simulink model "sedemo_mm1"  (Simulink 7.5)
settings: Solver=ode45  StartTime=0.0  StopTime=10000  RelTol=1e-3
PostLoadFcn:
  | open_system([gcs '/Arrival Rate Gain']);
undefined symbols (not defined in the file or in its folder): des_figposition, des_subsystemblock, des_subsysteminport, des_subsystemsupportblock
libraries: simeventssink1 x5, simulink x3, simeventstranslate1 x1, simeventsqueue1 x1, simeventsinfo x1, simeventsserver1 x1, simeventsgenerators1 x1
CloseFcn:
  | close_system([gcs '/Arrival Rate Gain']);
settings Model: Creator=The MathWorks Inc.  ExtModeAutoUpdateStatusClock=off
settings DataIOCC: SaveOutput=off  SaveTime=off
settings OptimizationCC: InlineInvariantSignals=on  InitFltsAndDblsToZero=on  BufferReusableBoundary=off
settings DebuggingCC: SignalResolutionControl=TryResolveAllWithWarning  SolverPrmCheckMsg=none  MultiTaskDSMMsg=warning  MultiTaskCondExecSysMsg=none  SigSpecEnsureSampleTimeMsg=none  BusObjectLabelMismatch=none  StrictBusMsg=None
settings RTWCC: IncludeERTFirstTime=on
settings SimEventsCC: propIdentEventSeed=12345678  propDiagAttribOutput=1  propDiagFcnCallOutput=1  propDiagStatOutput=0

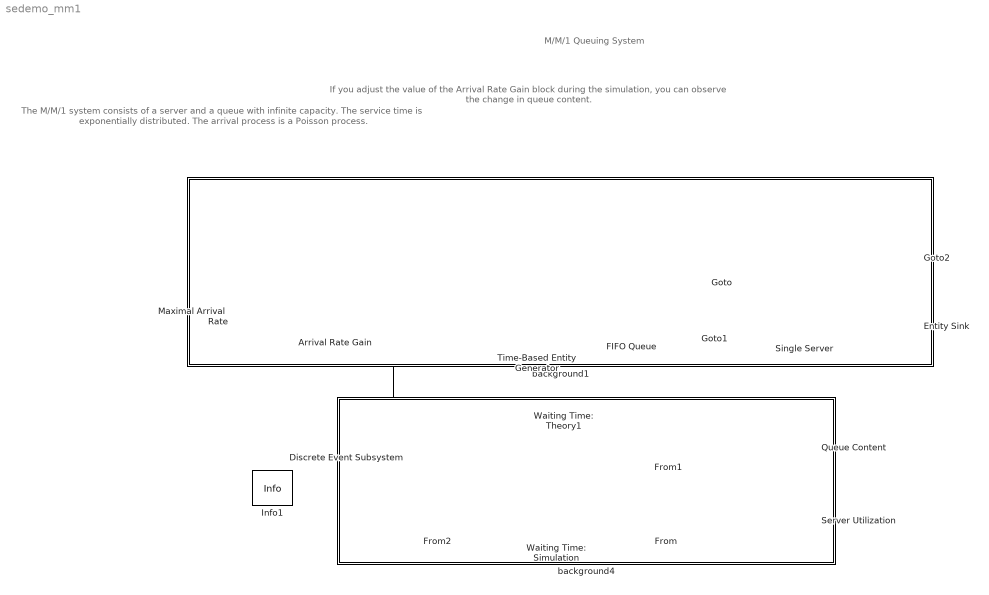
== system sedemo_mm1 ==
  note: M/M/1 Queuing System
  note: The M/M/1 system consists of a server
      | and a queue with infinite capacity. The
      | service time is exponentially distributed.
      | The arrival process is a Poisson process.
  note: If you adjust the value of the Arrival Rate Gain
      | block during the simulation, you can observe
      | the change in queue content.
  " " : Subsystem  mask(Exponential Random Number Generator){seed=96286}
      mask prompts: seed "Initial seed"
      mask help: Output exponentially distributed random numbers with rate 1. Output is repeatable for a given seed.
      mask Display: disp('Exponential\nDistribution\nwith Rate 1');
  "  " : Subsystem  mask(Exponential Random Number Generator){seed=85274}
      mask prompts: seed "Initial seed"
      mask help: Output exponentially distributed random numbers with the input rate. Output is repeatable for a given seed.
      mask Display: disp('Exponential\n Distribution');
  Arrival Rate Gain : simulink/Math Operations/Slider Gain  SystemSampleTime=-1  low=0.1  gain=0.5  high=0.999
  Discrete Event Subsystem : Subsystem  LoadFcn=des_subsystemblock(gcb, 'load');  InitFcn=des_subsystemblock(gcb, 'init');  StartFcn=des_subsystemblock(gcb, 'start');  StopFcn=des_subsystemblock(gcb, 'stop');
      settings: CopyFcn=des_subsystemblock(gcb, 'copy');  DeleteFcn=des_subsystemblock(gcb, 'delete');  UndoDeleteFcn=des_subsystemblock(gcb, 'undodelete');  ModelCloseFcn=des_subsystemblock(gcb, 'modelclose');  PreSaveFcn=des_subsystemblock(gcb, 'presave');  NameChangeFcn=des_subsystemblock(gcb, 'namechange');  OpenFcn=des_subsystemblock(gcb, 'open');  ParentCloseFcn=des_subsystemblock(gcb, 'parentclose');  ErrorFcn=des_subsystemerror
      mask Type: Discrete Event Subsystem
      mask Help: helpview(simeventsbhelp);
  Entity Sink : simeventssink1/Entity Sink  Priority=1  SystemSampleTime=-1  AvailableForArrivals=on  StatNumberArrived=Off
  FIFO Queue : simeventsqueue1/FIFO Queue  Priority=1  SystemSampleTime=-1  Capacity=Inf  EnableTOPort=off  StatNumberDeparted=Off  StatNumberInBlock=On  StatPendingEntity=Off  StatAverageWait=On  StatAverageQueueLength=Off  StatNumberTimedout=Off
  Info1 : simeventsinfo/Info  SystemSampleTime=-1
  Maximal Arrival  Rate : Constant  OutDataType=sfix(16)  OutScaling=2^0
  Queue Content : simeventssink1/Signal Scope  Priority=1  SystemSampleTime=-1  PlotType=Stair  InputType=Signal  NumInputs=1  AttributeNameY=Count  XInputOptionSignal=Event time  XInputOptionEntity=Event time  AttributeNameX=Count  EnableEntityOutport=on  XMin=0  XMax=Inf  XLimitExceededOption=Stretch axis limits  YLimitExceededOption=Stretch axis limits  AxisGrid=on  AxisLegend=off  LineDisables=""  LineColors=b  LineStyles=-  LineMarkers=.  OpenScopeAtSimStart=on  Title=Queue Content  YLabel=Queue Content  XLabel=Time  FigurePosition=des_figposition([47,5,22,22])  AxisZoom=off  DataStoreOption=Limited  DataPointsLimit=100000  StatNumberArrived=Off  ShowCountPlotted=off  ShowToolbar=off
      settings: YMin=0  YMax=Inf
  Server Utilization : simeventssink1/Signal Scope  Priority=1  SystemSampleTime=-1  PlotType=Stair  InputType=Signal  NumInputs=1  AttributeNameY=Count  XInputOptionSignal=Event time  XInputOptionEntity=Event time  AttributeNameX=Count  EnableEntityOutport=on  XMin=0  XMax=Inf  XLimitExceededOption=Stretch axis limits  YLimitExceededOption=Stretch axis limits  AxisGrid=on  AxisLegend=off  LineDisables=""  LineColors=b  LineStyles=-  LineMarkers=.  OpenScopeAtSimStart=on  Title=Server Utilization  YLabel=Utilization  XLabel=Time  FigurePosition=des_figposition([70,5,22,22])  AxisZoom=off  DataStoreOption=Limited  DataPointsLimit=100000  StatNumberArrived=Off  ShowCountPlotted=off  ShowToolbar=off
      settings: YMin=0  YMax=Inf
  Single Server : simeventsserver1/Single Server  Priority=1  SystemSampleTime=-1  ServiceTimeFrom=Signal port t  ServiceTime=1  AttributeName=ServiceTime  PriorityServiceCompletion=1  PermitPreemption=off  SortingAttributeName=PriorityAttributeName  SortingDirection=Ascending  WriteToAttribute=off  ResidualAttributeName=ResidualServiceTime  CreateAttribute=on  EnableTOPort=off  StatNumberDeparted=Off  StatNumberInBlock=Off  StatNumberPreempted=Off  StatPendingEntity=Off  StatAverageWait=Off  StatUtilization=On  StatNumberTimedout=Off
  Time-Based Entity Generator : simeventsgenerators1/Entity Generators/Time-Based Entity Generator  Priority=1  DialogController=des_ddg_create  DialogControllerArgs=DataTag13  SystemSampleTime=-1  GenerateEntitiesUpon=Intergeneration time from port t  Distribution=Constant  Minimum=0  Maximum=1  Mean=1  InitialSeed=12345  Period=1  PriorityEntityGeneration=1  GenerateEntityAtSimulationStart=on  ResponseWhenBlocked=Error  ResponseWhenUnblocked=Immediate restart  EntityType=Standard  StatNumberDeparted=Off  StatPendingEntity=Off  StatAverageIntergenerationTime=Off
  Waiting Time: Simulation : simeventssink1/Signal Scope  Priority=1  SystemSampleTime=-1  PlotType=Continuous  InputType=Signal  NumInputs=1  AttributeNameY=Count  XInputOptionSignal=Event time  XInputOptionEntity=Event time  AttributeNameX=Count  EnableEntityOutport=on  XMin=0  XMax=Inf  XLimitExceededOption=Stretch axis limits  YLimitExceededOption=Stretch axis limits  AxisGrid=on  AxisLegend=off  LineDisables=""  LineColors=b  LineStyles=-  LineMarkers=.  OpenScopeAtSimStart=on  Title=Waiting Time: Simulation  YLabel=Waiting Time  XLabel=Time  FigurePosition=des_figposition([23,5,22,22])  AxisZoom=off  DataStoreOption=Limited  DataPointsLimit=100000  StatNumberArrived=Off  ShowCountPlotted=on  ShowToolbar=off
      settings: YMin=0  YMax=Inf
  Waiting Time: Theory1 : simeventssink1/Signal Scope  Priority=1  SystemSampleTime=-1  PlotType=Continuous  InputType=Signal  NumInputs=1  AttributeNameY=Count  XInputOptionSignal=Event time  XInputOptionEntity=Event time  AttributeNameX=Count  EnableEntityOutport=on  XMin=0  XMax=10240  XLimitExceededOption=Stretch axis limits  YLimitExceededOption=Stretch axis limits  AxisGrid=on  AxisLegend=off  LineDisables=""  LineColors=b  LineStyles=-  LineMarkers=.  OpenScopeAtSimStart=on  Title=Waiting Time : Theory  YLabel=Waiting Time  XLabel=Time  FigurePosition=des_figposition([0,5,22,22])  AxisZoom=off  DataStoreOption=Limited  DataPointsLimit=10000  StatNumberArrived=Off  ShowCountPlotted=on  ShowToolbar=off
      settings: YMin=0  YMax=3
  background1 : Subsystem
      mask Display: disp('')
  background4 : Subsystem
      mask Display: disp('')
  wires:
  " "/1("Service Time ") -> Single Server/1
  Maximal Arrival  Rate/1 -> Arrival Rate Gain/1
  Discrete Event Subsystem/1(Dout1) -> Waiting Time: Theory1/1
  "  "/1(Out1) -> Time-Based Entity Generator/1
  Arrival Rate Gain/1 -> "  "/1(Arrival Rate), Discrete Event Subsystem/1(Arrival Rate)
  [Ser_util] -> Server Utilization/1
  [Q_n] -> Queue Content/1
  [Q_w] -> Waiting Time: Simulation/1
  FIFO Queue/1 -> [Q_n]
  FIFO Queue/2 -> [Q_w]
  Single Server/1 -> [Ser_util]
  connections:
  Time-Based Entity Generator/RConn1 -- FIFO Queue/LConn1
  FIFO Queue/RConn1 -- Single Server/LConn1
  Single Server/RConn1 -- Entity Sink/LConn1

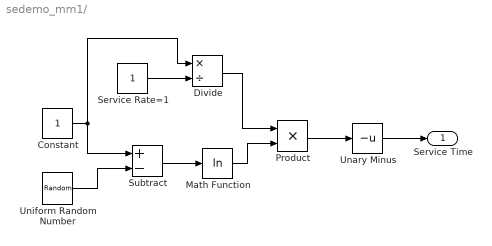
== system sedemo_mm1/  ==
  Constant : Constant  OutDataType=sfix(16)  OutScaling=2^0
  Divide : Product  Inputs=*/  OutDataType=sfix(16)  OutScaling=2^-10
  Math Function : Math  Operator=log  OutDataType=sfix(16)  OutScaling=2^0  SaturateOnIntegerOverflow=on
  Product : Product  OutDataType=sfix(16)  OutScaling=2^0  RndMeth=Zero
  Service Rate=1 : Constant  OutDataType=sfix(16)  OutScaling=2^0
  Subtract : Sum  Inputs=+-  OutDataType=sfix(16)  OutScaling=2^-10
  Unary Minus : UnaryMinus
  Uniform Random Number : UniformRandomNumber  Minimum=0  Seed=seed  SampleTime=0
  "Service Time " : Outport  OutDataType=sfix(16)  OutScaling=2^0
  wires:
  Divide/1 -> Product/1
  Service Rate=1/1 -> Divide/2
  Constant/1 -> Divide/1, Subtract/1
  Uniform Random Number/1 -> Subtract/2
  Subtract/1 -> Math Function/1
  Math Function/1 -> Product/2
  Product/1 -> Unary Minus/1
  Unary Minus/1 -> "Service Time "/1

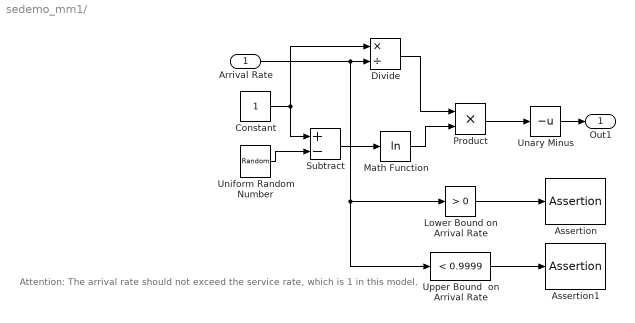
== system sedemo_mm1/   ==
  note: Attention: The arrival rate
      | should not exceed the service
      | rate, which is 1 in this model.
  Arrival Rate : Inport  OutDataType=sfix(16)  OutScaling=2^0
  Assertion : Assertion  Enabled=on
  Assertion1 : Assertion  Enabled=on
  Constant : Constant  OutDataType=sfix(16)  OutScaling=2^0
  Divide : Product  Inputs=*/  OutDataType=sfix(16)  OutScaling=2^-10
  Lower Bound on Arrival Rate : simulink/Logic and Bit Operations/Compare To Constant  SystemSampleTime=-1  relop=>  const=0  LogicOutDataTypeMode=uint8  ZeroCross=off
  Math Function : Math  Operator=log  OutDataType=sfix(16)  OutScaling=2^0  SaturateOnIntegerOverflow=on
  Product : Product  OutDataType=sfix(16)  OutScaling=2^0  RndMeth=Zero
  Subtract : Sum  Inputs=+-  OutDataType=sfix(16)  OutScaling=2^-10
  Unary Minus : UnaryMinus
  Uniform Random Number : UniformRandomNumber  Minimum=0  Seed=seed  SampleTime=0
  "Upper Bound  on Arrival Rate " : simulink/Logic and Bit Operations/Compare To Constant  SystemSampleTime=-1  relop=<  const=0.9999  LogicOutDataTypeMode=uint8  ZeroCross=off
  Out1 : Outport  OutDataType=sfix(16)  OutScaling=2^0
  wires:
  Unary Minus/1 -> Out1/1
  Product/1 -> Unary Minus/1
  Math Function/1 -> Product/2
  Subtract/1 -> Math Function/1
  Uniform Random Number/1 -> Subtract/2
  Constant/1 -> Subtract/1, Divide/1
  Arrival Rate/1 -> Divide/2, Lower Bound on Arrival Rate/1, "Upper Bound  on Arrival Rate "/1
  Divide/1 -> Product/1
  Lower Bound on Arrival Rate/1 -> Assertion/1
  "Upper Bound  on Arrival Rate "/1 -> Assertion1/1

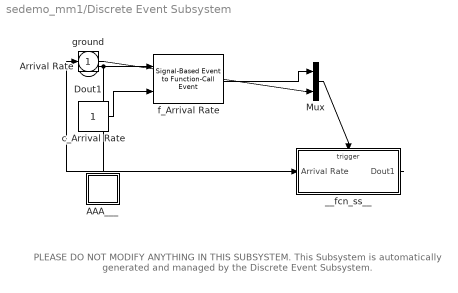
== system sedemo_mm1/Discrete Event Subsystem ==
  note: PLEASE DO NOT MODIFY ANYTHING IN THIS SUBSYSTEM.
      | This Subsystem is automatically generated and
      | managed by the Discrete Event Subsystem.
  Arrival Rate : Inport  DataType=double  OutDataType=sfix(16)  OutScaling=2^0  OutDataTypeStr=double
  AAA___ : Subsystem  LoadFcn=des_subsystemsupportblock(gcb, 'load');  InitFcn=des_subsystemsupportblock(gcb, 'init');  StartFcn=des_subsystemsupportblock(gcb, 'start');  StopFcn=des_subsystemsupportblock(gcb, 'stop');
      settings: CopyFcn=des_subsystemsupportblock(gcb, 'copy');  DeleteFcn=des_subsystemsupportblock(gcb, 'delete');  UndoDeleteFcn=des_subsystemsupportblock(gcb, 'undodelete');  ModelCloseFcn=des_subsystemsupportblock(gcb, 'modelclose');  PreSaveFcn=des_subsystemsupportblock(gcb, 'presave');  NameChangeFcn=des_subsystemsupportblock(gcb, 'namechange');  OpenFcn=des_subsystemsupportblock(gcb, 'open');  ParentCloseFcn=des_subsystemsupportblock(gcb, 'parentclose');
  Mux : Mux  Inputs=2
  __fcn_ss__ : Subsystem  TreatAsAtomicUnit=on
      settings: PropExecContextOutsideSubsystem=on
  c_Arrival Rate : Constant  OutDataType=sfix(16)  OutScaling=2^0
  f_Arrival Rate : simeventstranslate1/Signal-Based Event to Function-Call Event  Priority=1  SystemSampleTime=-1  GenerateFunctionCallUpon=Sample time hit from port ts  SignalEdgeOption=Rising  EnableE1Port=on  EnableF2Port=off  EnableE2Port=off  SpecifyEventPriority=off  PriorityFunctionCall=20  FunctionCallDelayFrom=Dialog  DelayFunctionCall=0  StatNumberF1Calls=Off  StatNumberF2Calls=Off  MaskBlockType=DESS_EVENT_PORT
  ground : Ground
  Dout1 : Outport  OutDataType=sfix(16)  OutScaling=2^0
  wires:
  f_Arrival Rate/1 -> Mux/1
  c_Arrival Rate/1 -> f_Arrival Rate/2
  Mux/1 -> __fcn_ss__/Trigger
  ground/1 -> Mux/2
  __fcn_ss__/1(Dout1) -> Dout1/1
  Arrival Rate/1 -> f_Arrival Rate/1, __fcn_ss__/1(Arrival Rate)

== system sedemo_mm1/background1 ==

== system sedemo_mm1/background4 ==

== system sedemo_mm1/Discrete Event Subsystem/AAA___ ==

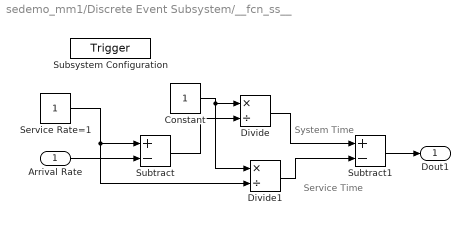
== system sedemo_mm1/Discrete Event Subsystem/__fcn_ss__ ==
  note: System Time
  note: Service Time
  Arrival Rate : Inport  LoadFcn=des_subsysteminport(gcb, 'load');  InitFcn=des_subsysteminport(gcb, 'init');  StartFcn=des_subsysteminport(gcb, 'start');  StopFcn=des_subsysteminport(gcb, 'stop');  OutDataType=sfix(16)  OutScaling=2^0  mask(Discrete Event Inport){PermitSubsystemEvents=on, TypeOfEvent=Sample time hit, SignalEdgeOption=Rising, SpecifyEventPriority=off, PrioritySubsystemEvent=20}
      mask prompts: PermitSubsystemEvents "Execute subsystem upon signal-based events"; TypeOfEvent "Type of signal-based event:"; SignalEdgeOption "Type of change in signal value:"; SpecifyEventPriority "Specify event priority for executing subsystem"; PrioritySubsystemEvent "Subsystem execution event priority:"
      mask help: Input port for a Discrete Event Subsystem block. This block can conditionally execute the subsystem upon signal-based events that meet specified criteria.
      mask init:
      | des_subsystemmask(gcb, 'init','apply')
      settings: CopyFcn=des_subsysteminport(gcb, 'copy');  DeleteFcn=des_subsysteminport(gcb, 'delete');  UndoDeleteFcn=des_subsysteminport(gcb, 'undodelete');  ModelCloseFcn=des_subsysteminport(gcb, 'modelclose');  PreSaveFcn=des_subsysteminport(gcb, 'presave');  NameChangeFcn=des_subsysteminport(gcb, 'namechange');  ParentCloseFcn=des_subsysteminport(gcb, 'parentclose');
      mask Help: helpview(simeventsbhelp);
      mask StyleString: checkbox,popup(Change in signal|Trigger|Sample time hit),popup(Rising|Falling|Either),checkbox,edit
      mask CallbackString: des_subsystemmask(gcb, 'cbPermitSubsystemEvents', 'noapply');|des_subsystemmask(gcb,'cbTypeOfEvent','noapply');||des_subsystemmask(gcb, 'cbSpecifyEventPriority', 'noapply');|
  Subsystem Configuration : TriggerPort  TriggerType=function-call
      settings: CopyFcn=des_subsystemconfigblock(gcb, 'copy');  DeleteFcn=des_subsystemconfigblock(gcb, 'delete');  UndoDeleteFcn=des_subsystemconfigblock(gcb, 'undodelete');
      mask Type: Subsystem Configuration
      mask Description: Configuration for a Discrete Event Subsystem block. Every discrete event subsystem window must contain exactly one copy of this configuration block. Do not delete this block.
      mask Help: helpview(simeventsbhelp);
      mask Display: disp('Do Not Delete');
  Constant : Constant  OutDataType=sfix(16)  OutScaling=2^0
  Divide : Product  Inputs=*/  OutDataType=sfix(16)  OutScaling=2^-10
  Divide1 : Product  Inputs=*/  OutDataType=sfix(16)  OutScaling=2^-10
  Service Rate=1 : Constant  OutDataType=sfix(16)  OutScaling=2^0
  Subtract : Sum  Inputs=+-  OutDataType=sfix(16)  OutScaling=2^-10
  Subtract1 : Sum  Inputs=+-  OutDataType=sfix(16)  OutScaling=2^-10
  Dout1 : Outport  OutDataType=sfix(16)  OutScaling=2^0
      settings: CopyFcn=des_subsystemconfig(gcb, 'copy', '');  DeleteFcn=des_subsystemconfig(gcb, 'delete', '');  UndoDeleteFcn=des_subsystemconfig(gcb, 'undodelete', '');  ModelCloseFcn=des_subsystemconfig(gcb, 'modelclose', '');  NameChangeFcn=des_subsystemconfig(gcb, 'namechange', '');
      mask Type: Discrete Event Outport
      mask Description: Provide an output port for a Discrete Event Subsystem block.
  wires:
  Service Rate=1/1 -> Subtract/1, Divide1/2
  Arrival Rate/1 -> Subtract/2
  Constant/1 -> Divide/1, Divide1/1
  Subtract/1 -> Divide/2
  Divide/1 -> Subtract1/1
  Divide1/1 -> Subtract1/2
  Subtract1/1 -> Dout1/1
